simulink library "Lib_Turbo_Bleed_TMATS"  (R2015a)
settings: Solver=ode45  StartTime=0.0  StopTime=10.0  RelTol=1e-3
Description:
  | Thomas Modules
settings Model: Creator=jwchapm2  LastModifiedBy=jwchapm2
settings OptimizationCC: ExpressionDepthLimit=2147483647
settings DebuggingCC: UnderspecifiedInitializationDetection=Classic  MergeDetectMultiDrivingBlocksExec=none  SolverPrmCheckMsg=warning  StateNameClashWarn=warning

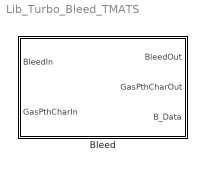
== system Lib_Turbo_Bleed_TMATS ==
  Bleed : Subsystem  TreatAsAtomicUnit=on  mask(T-MATS: Bleed Library Block){Wfrac_M=[0], BlkNm_M=0}
      mask prompts: Wfrac_M "Wfrac_M - Output Bleed Fractions[frac](1xn)"; BlkNm_M "Block name as double for Simulink output"
      mask help: This block extracts bleed flows from the main stream or combines flows into the main stream. It should be noted that this block is meant for small bleed flows. Inflows are introduced to the main flow as to preserve total mass flow and total enthalpy, however momentum calculations are not performed. Outflows are defined fractionally based on the main input flow.
      mask Help: web(which('Turbo_TMATS_Bld.html'),'-helpbrowser')

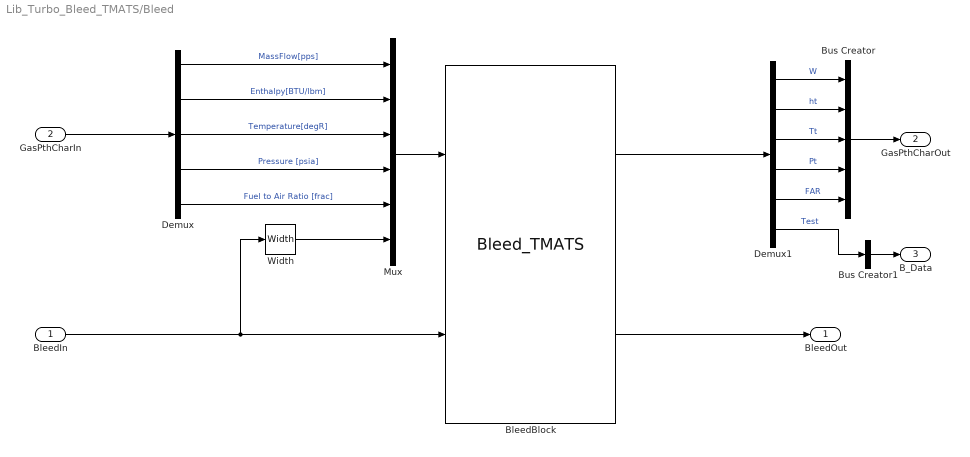
== system Lib_Turbo_Bleed_TMATS/Bleed ==
  BleedIn : Inport
  GasPthCharIn : Inport  Port=2
  BleedBlock : S-Function  FunctionName=Bleed_TMATS  Parameters=Wfrac_M ,length(Wfrac_M),BlkNm_M  SFunctionModules='h2tc_TMATS t2hc_TMATS functions_TMATS'
  Bus Creator : BusCreator  Inputs=5
  Bus Creator1 : BusCreator  Inputs=1
  Demux : Demux  Outputs=5
  Demux1 : Demux  Outputs=6
  Mux : Mux  Inputs=6
  Width : Width
  BleedOut : Outport  PortDimensions=5*length(Wfrac_M)
  GasPthCharOut : Outport  Port=2
  B_Data : Outport  Port=3
  wires:
  BleedBlock/1 -> Demux1/1
  Mux/1 -> BleedBlock/1
  Demux/3 -> Mux/3  "Temperature[degR]"
  Demux/5 -> Mux/5  "Fuel to Air Ratio [frac]"
  Demux/4 -> Mux/4  "Pressure [psia]"
  GasPthCharIn/1 -> Demux/1
  BleedIn/1 -> Width/1, BleedBlock/2
  Demux/1 -> Mux/1  "MassFlow[pps]"
  Demux/2 -> Mux/2  "Enthalpy[BTU/lbm]"
  Width/1 -> Mux/6
  BleedBlock/2 -> BleedOut/1
  Bus Creator/1 -> GasPthCharOut/1
  Demux1/2 -> Bus Creator/2  "ht"
  Demux1/1 -> Bus Creator/1  "W"
  Demux1/5 -> Bus Creator/5  "FAR"
  Demux1/4 -> Bus Creator/4  "Pt"
  Demux1/3 -> Bus Creator/3  "Tt"
  Demux1/6 -> Bus Creator1/1  "Test"
  Bus Creator1/1 -> B_Data/1
